simulink model "ALS"  (R2012b)
settings: Solver=ode1  StartTime=0.0  StopTime=200  FixedStep=0.05  RelTol=1e-3
undefined symbols (not defined in the file or in its folder): ACSP
libraries: simulink x2
settings Model: BufferReuse=off  Creator=jmbianni  LastModifiedBy=biannic
settings DataIOCC: InitialState=[]  LoadInitialState=on
settings OptimizationCC: InlineParams=on  BufferReuse=off
settings DebuggingCC: InitInArrayFormatMsg=none
settings CodeAppCC: CustomSymbolStrType=$N$R$M_T
settings GRTTargetCC: CodeReplacementLibrary=C89/C90 (ANSI)

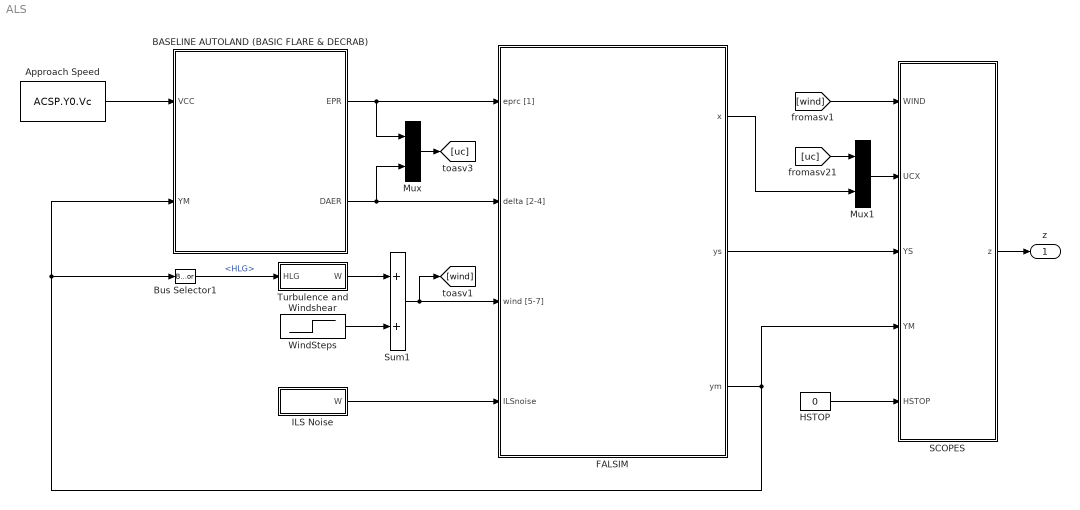
== system ALS ==
  Approach Speed : Constant  Value=ACSP.Y0.Vc
  BASELINE AUTOLAND (BASIC FLARE & DECRAB) : Subsystem
      mask Display:
      | image(imread('ALS.png'));
      | 
      | port_label('output', 1,'{\bf\fontsize{12}\delta_{TH}}', 'texmode','on');
      | port_label('output', 2,'{\bf\fontsize{12}\delta_{AER}}', 'texmode','on');
      | port_label('input', 1,'{\bf\fontsize{12}V_{APP}}', 'texmode','on');
      | port_label('input', 2,'{\bf\fontsize{12}YM}', 'texmode','on');
  Bus Selector1 : BusSelector  OutputSignals=HLG
  FALSIM : Subsystem
      mask Display:
      | image(imread('FALSIM.png'));
      | color('white');
      | disp('FINAL APPROACH & LANDING \n\n\n\n\n\n\n\n\n\n\n\n\n\n\n\n\n\n\n\n\n\n\n\n\n\n\n\n\n\n');
      | disp('SIMULATION MODEL \n\n\n\n\n\n\n\n\n\n\n\n\n\n\n\n\n\n\n\n\n\n\n\n\n\n\n\n');
      | 
      | color('red');
      | disp('http://w3.onera.fr/smac/ \n\n\n\n');
      | 
      | 
      | 
      | color('red');
      | %disp('{\bf\fontsize{12}SMAC TOOLS}', 'texmode','on');
      | 
      | color('yellow');
      | 
      | port_label('output', 1,'{\bf\fontsize{12}States}', 'texmode','on');
      | port_label('output', 2,'{\bf\fontsize{12}Non Measured Outputs}', 'texmode','on');
      | port_label('output', 3,'{\bf\fontsize{12}Measured Outputs}', 'texmode','on');
      | port_label('input', 1,'{\bf\fontsize{12}\delta_{TH}}', 'texmode','on');
      | port_label('input', 2,'{\bf\fontsize{12}\delta_A , \delta_E , \delta_R}', 'texmode','on');
      | port_label('input', 3,'{\bf\fontsize{12}W_x , W_y , W_z}', 'texmode','on');
      | port_label('input', 4,'{\bf\fontsize{12}W_{LOC} , W_{GLD}}', 'texmode','on');
  HSTOP : Constant  Value=0
  ILS Noise : Subsystem
  Mux : Mux  Inputs=2
  Mux1 : Mux  Inputs=2
  SCOPES : Subsystem
  Sum1 : Sum
  Turbulence and Windshear : Subsystem
  WindSteps : Step  Time=ACSP.TURBW.WindStepTime  After=ACSP.TURBW.WindStepMag  SampleTime=0
  z : Outport
  wires:
  BASELINE AUTOLAND (BASIC FLARE & DECRAB)/1(EPR) -> FALSIM/1(eprc [1]), Mux/1
  BASELINE AUTOLAND (BASIC FLARE & DECRAB)/2(DAER) -> FALSIM/2(delta [2-4]), Mux/2
  FALSIM/3(ym) -> SCOPES/4(YM), BASELINE AUTOLAND (BASIC FLARE & DECRAB)/2(YM), Bus Selector1/1
  Approach Speed/1 -> BASELINE AUTOLAND (BASIC FLARE & DECRAB)/1(VCC)
  SCOPES/1(z) -> z/1
  Mux/1 -> [uc]
  FALSIM/1(x) -> Mux1/2
  [uc] -> Mux1/1
  FALSIM/2(ys) -> SCOPES/3(YS)
  Mux1/1 -> SCOPES/2(UCX)
  HSTOP/1 -> SCOPES/5(HSTOP)
  Bus Selector1/1 -> Turbulence and Windshear/1(HLG)  "<HLG>"
  ILS Noise/1(W) -> FALSIM/4(ILSnoise)
  [wind] -> SCOPES/1(WIND)
  Sum1/1 -> FALSIM/3(wind [5-7]), [wind]
  Turbulence and Windshear/1(W) -> Sum1/1
  WindSteps/1 -> Sum1/2

== system ALS/BASELINE AUTOLAND (BASIC FLARE & DECRAB) ==
  VCC : Inport
  YM : Inport  Port=2
  DECRAB : Subsystem
  FLARE : Subsystem
  GLD  OUTER-LOOP : Subsystem
  HDEC : Constant  Value=ACSP.ALS.HDC
  HFLA : Constant  Value=ACSP.ALS.HFL
  LAT CONTROL : Subsystem
  LOC OUTER-LOOP : Subsystem
  LON CONTROL : Subsystem
  Mux : Mux  Inputs=2
  Switch DEC : Switch
  Switch FLA : Switch
  dth1 : Selector  InputPortWidth=4  IndexOptions=Index vector (dialog)  Indices=1  OutputSizes=1
  dth2 : Selector  InputPortWidth=4  IndexOptions=Index vector (dialog)  Indices=[3 2 4]  OutputSizes=1
  EPR : Outport
  DAER : Outport  Port=2
  wires:
  FLARE/2(dTH dE) -> Switch FLA/3
  FLARE/1(swF) -> Switch FLA/2
  HDEC/1 -> DECRAB/2(HDEC)
  dth2/1 -> DAER/1
  dth1/1 -> EPR/1
  Mux/1 -> dth2/1, dth1/1
  HFLA/1 -> FLARE/2(HFL)
  LON CONTROL/1(dTH  dE) -> Switch FLA/1, FLARE/1(dTHdE)
  Switch FLA/1 -> Mux/1
  DECRAB/1(swD) -> Switch DEC/2
  DECRAB/2(nyc,phic) -> Switch DEC/3
  Switch DEC/1 -> LAT CONTROL/2(nyc,phic)
  LOC OUTER-LOOP/1(nyc,phic) -> Switch DEC/1
  VCC/1 -> GLD  OUTER-LOOP/1(Vcc)
  LAT CONTROL/1(dA  dR) -> Mux/2
  GLD  OUTER-LOOP/1(vcc,vzc) -> LON CONTROL/1(vcc,vzc)
  YM/1 -> GLD  OUTER-LOOP/2(y), LON CONTROL/2(y), LAT CONTROL/1(y), FLARE/3(y), DECRAB/1(y), LOC OUTER-LOOP/1(y)

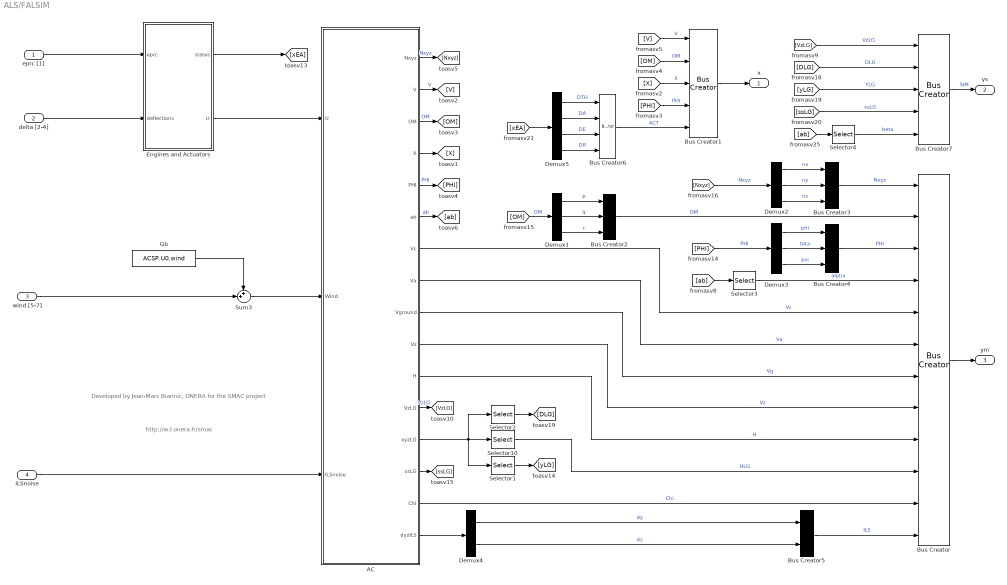
== system ALS/FALSIM ==
  note: http://w3.onera.fr/smac
  note: Developed by
      | Jean-Marc Biannic, ONERA
      | for the SMAC project
  eprc [1] : Inport
  delta [2-4] : Inport  Port=2  PortDimensions=3
  wind [5-7] : Inport  Port=3  PortDimensions=3
  ILSnoise : Inport  Port=4  PortDimensions=2
  AC : Subsystem
  Bus Creator : BusCreator  Inputs=12
  Bus Creator1 : BusCreator  Inputs=5
  Bus Creator2 : BusCreator  Inputs=3
  Bus Creator3 : BusCreator  Inputs=3
  Bus Creator4 : BusCreator  Inputs=3
  Bus Creator5 : BusCreator  Inputs=2
  Bus Creator6 : BusCreator
  Bus Creator7 : BusCreator  Inputs=5
  Demux1 : Demux  Outputs=3
  Demux2 : Demux  Outputs=3
  Demux3 : Demux  Outputs=3
  Demux4 : Demux  Outputs=2
  Demux5 : Demux
  Engines and Actuators : Subsystem
  Gb : Constant  Value=ACSP.U0.wind
  Selector1 : Selector  InputPortWidth=3  IndexOptions=Index vector (dialog)  Indices=2  OutputSizes=1
  Selector10 : Selector  InputPortWidth=3  IndexOptions=Index vector (dialog)  Indices=3  OutputSizes=1
  Selector2 : Selector  InputPortWidth=3  IndexOptions=Index vector (dialog)  Indices=1  OutputSizes=1
  Selector3 : Selector  InputPortWidth=2  IndexOptions=Index vector (dialog)  Indices=1  OutputSizes=1
  Selector4 : Selector  InputPortWidth=2  IndexOptions=Index vector (dialog)  Indices=2  OutputSizes=1
  Sum3 : Sum  Inputs=++|
  x : Outport
  ys : Outport  Port=2
  ym : Outport  Port=3
  wires:
  [VzLG] -> Bus Creator7/1  "VzLG"
  [DLG] -> Bus Creator7/2  "DLG"
  [yLG] -> Bus Creator7/3  "YLG"
  [ssLG] -> Bus Creator7/4  "ssLG"
  Selector4/1 -> Bus Creator7/5  "beta"
  delta [2-4]/1 -> Engines and Actuators/2(deflections)
  Bus Creator7/1 -> ys/1  "SIM"
  Bus Creator/1 -> ym/1
  Sum3/1 -> AC/2(Wind)
  Gb/1 -> Sum3/1
  ILSnoise/1 -> AC/3(ILSnoise)
  AC/11(H) -> Bus Creator/9  "H"
  AC/10(Vz) -> Bus Creator/8  "Vz"
  [ab] -> Selector4/1
  Bus Creator5/1 -> Bus Creator/12  "ILS"
  Bus Creator6/1 -> Bus Creator1/5  "ACT"
  [xEA] -> Demux5/1
  Demux5/4 -> Bus Creator6/4  "DR"
  Demux5/3 -> Bus Creator6/3  "DE"
  Demux5/2 -> Bus Creator6/2  "DA"
  Demux5/1 -> Bus Creator6/1  "DTH"
  Engines and Actuators/1(states) -> [xEA]
  Engines and Actuators/2(U) -> AC/1(U)
  eprc [1]/1 -> Engines and Actuators/1(eprc)
  Bus Creator1/1 -> x/1
  [PHI] -> Bus Creator1/4  "PHI"
  [X] -> Bus Creator1/3  "X"
  [OM] -> Bus Creator1/2  "OM"
  [V] -> Bus Creator1/1  "V"
  AC/12(VzLG) -> [VzLG]  "VzLG"
  AC/15(Chi) -> Bus Creator/11  "Chi"
  AC/9(Vground) -> Bus Creator/7  "Vg"
  AC/8(Va) -> Bus Creator/6  "Va"
  AC/7(Vc) -> Bus Creator/5  "Vc"
  AC/6(ab) -> [ab]  "ab"
  AC/5(PHI) -> [PHI]  "PHI"
  AC/4(X) -> [X]
  AC/3(OM) -> [OM]  "OM"
  AC/2(V) -> [V]  "V"
  AC/1(Nxyz) -> [Nxyz]  "Nxyz"
  Selector10/1 -> Bus Creator/10  "HLG"
  Selector2/1 -> [DLG]
  Demux4/2 -> Bus Creator5/2  "dz"
  Demux4/1 -> Bus Creator5/1  "dy"
  AC/16(dyzILS) -> Demux4/1
  AC/14(ssLG) -> [ssLG]
  Selector1/1 -> [yLG]
  AC/13(xyzLG) -> Selector2/1, Selector10/1, Selector1/1
  Bus Creator4/1 -> Bus Creator/3  "PHI"
  [PHI] -> Demux3/1  "PHI"
  Demux3/1 -> Bus Creator4/1  "phi"
  Demux3/2 -> Bus Creator4/2  "teta"
  Demux3/3 -> Bus Creator4/3  "psi"
  Bus Creator3/1 -> Bus Creator/1  "Nxyz"
  [Nxyz] -> Demux2/1  "Nxyz"
  Demux2/1 -> Bus Creator3/1  "nx"
  Demux2/2 -> Bus Creator3/2  "ny"
  Demux2/3 -> Bus Creator3/3  "nz"
  [OM] -> Demux1/1  "OM"
  Demux1/1 -> Bus Creator2/1  "p"
  Demux1/2 -> Bus Creator2/2  "q"
  Demux1/3 -> Bus Creator2/3  "r"
  Bus Creator2/1 -> Bus Creator/2  "OM"
  [ab] -> Selector3/1
  Selector3/1 -> Bus Creator/4  "alpha"
  wind [5-7]/1 -> Sum3/2

== system ALS/ILS Noise ==
  Mux : Mux  Inputs=2
  Random Number : RandomNumber  Seed=ACSP.NOISE.seedLOC  SampleTime=0.05
  Random Number3 : RandomNumber  Seed=ACSP.NOISE.seedGLD  SampleTime=0.05
  Sum12 : Sum  Inputs=++|
  bias : Constant  Value=ACSP.NOISE.devLOC
  sigGLD : Gain  Gain=ACSP.NOISE.sigGLD
  sigLOC : Gain  Gain=ACSP.NOISE.sigLOC
  srqt(2*tau/ts)*1/(1+tau.s) : TransferFcn  Numerator=[4.5]  Denominator=[0.5 1]
  srqt(2*tau/ts)*1/(1+tau.s)1 : TransferFcn  Numerator=[4.5]  Denominator=[0.5 1]
  W : Outport
  wires:
  bias/1 -> Sum12/1
  Sum12/1 -> Mux/1
  sigLOC/1 -> Sum12/2
  sigGLD/1 -> Mux/2
  srqt(2*tau/ts)*1/(1+tau.s)/1 -> sigLOC/1
  Random Number3/1 -> srqt(2*tau/ts)*1/(1+tau.s)1/1
  Random Number/1 -> srqt(2*tau/ts)*1/(1+tau.s)/1
  Mux/1 -> W/1
  srqt(2*tau/ts)*1/(1+tau.s)1/1 -> sigGLD/1

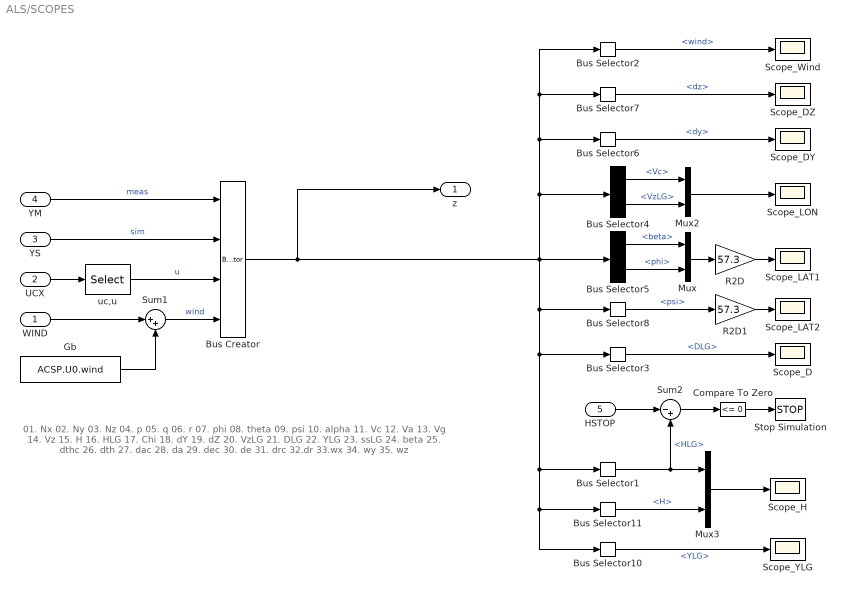
== system ALS/SCOPES ==
  note: 01. Nx       02. Ny        03. Nz         04. p         05. q         06. r        07. phi         08. theta           09. psi
      | 10. alpha        11. Vc       12. Va      13. Vg       14. Vz        15. H        16. HLG       17. Chi     18. dY
      | 19. dZ     20. VzLG         21. DLG     22. YLG    23. ssLG      24. beta       25. dthc      26. dth
      |  27. dac        28. da          29. dec          30. de          31.  drc        32.dr        33.wx      34. wy    35. wz
  WIND : Inport
  UCX : Inport  Port=2
  YS : Inport  Port=3
  YM : Inport  Port=4
  HSTOP : Inport  Port=5
  Bus Creator : BusCreator
  Bus Selector1 : BusSelector  OutputSignals=meas.HLG
  Bus Selector10 : BusSelector  OutputSignals=sim.YLG
  Bus Selector11 : BusSelector  OutputSignals=meas.H
  Bus Selector2 : BusSelector  OutputSignals=wind
  Bus Selector3 : BusSelector  OutputSignals=sim.DLG
  Bus Selector4 : BusSelector  OutputSignals=meas.Vc,sim.VzLG
  Bus Selector5 : BusSelector  OutputSignals=sim.beta,meas.PHI.phi
  Bus Selector6 : BusSelector  OutputSignals=meas.ILS.dy
  Bus Selector7 : BusSelector  OutputSignals=meas.ILS.dz
  Bus Selector8 : BusSelector  OutputSignals=meas.PHI.psi
  Compare To Zero : simulink/Logic and Bit Operations/Compare To Zero  relop=<=  OutDataTypeStr=boolean
  Gb : Constant  Value=ACSP.U0.wind
  Mux : Mux  Inputs=2
  Mux2 : Mux  Inputs=2
  Mux3 : Mux  Inputs=2
  R2D : Gain  Gain=57.3
  R2D1 : Gain  Gain=57.3
  Scope_D : Scope
      settings: SaveName=ScopeData9
  Scope_DY : Scope
  Scope_DZ : Scope
      settings: SaveName=ScopeData2  Decimation=2
  Scope_H : Scope
      settings: SaveName=ScopeData3  Decimation=2
  Scope_LAT1 : Scope
      settings: SaveName=ScopeData4
  Scope_LAT2 : Scope
  Scope_LON : Scope
      settings: SaveName=ScopeData5
  Scope_Wind : Scope
      settings: SaveName=ScopeData8  Decimation=2
  Scope_YLG : Scope
      settings: YMin=2.5  YMax=22.5  SaveName=ScopeData6  Decimation=2
  Stop Simulation : Stop
  Sum1 : Sum  Inputs=|++
  Sum2 : Sum  Inputs=|-+
  uc,u : Selector  InputPortWidth=20  IndexOptions=Index vector (dialog)  Indices=[1 17 2 18 3 19 4 20]  OutputSizes=1
  z : Outport
  wires:
  Bus Selector10/1 -> Scope_YLG/1  "<YLG>"
  Mux3/1 -> Scope_H/1
  Bus Selector3/1 -> Scope_D/1  "<DLG>"
  R2D1/1 -> Scope_LAT2/1
  Bus Selector8/1 -> R2D1/1  "<psi>"
  R2D/1 -> Scope_LAT1/1
  Mux/1 -> R2D/1
  Mux2/1 -> Scope_LON/1
  Bus Selector4/2 -> Mux2/2  "<VzLG>"
  Bus Selector4/1 -> Mux2/1  "<Vc>"
  YM/1 -> Bus Creator/1  "meas"
  Bus Selector7/1 -> Scope_DZ/1  "<dz>"
  Bus Selector6/1 -> Scope_DY/1  "<dy>"
  YS/1 -> Bus Creator/2  "sim"
  Bus Selector1/1 -> Sum2/2, Mux3/1  "<HLG>"
  Bus Selector11/1 -> Mux3/2  "<H>"
  Bus Creator/1 -> Bus Selector2/1, Bus Selector7/1, Bus Selector6/1, Bus Selector4/1, Bus Selector10/1, Bus Selector11/1, Bus Selector1/1, Bus Selector3/1, Bus Selector8/1, Bus Selector5/1, z/1
  uc,u/1 -> Bus Creator/3  "u"
  Bus Selector5/2 -> Mux/2  "<phi>"
  UCX/1 -> uc,u/1
  Bus Selector5/1 -> Mux/1  "<beta>"
  Compare To Zero/1 -> Stop Simulation/1
  Sum2/1 -> Compare To Zero/1
  HSTOP/1 -> Sum2/1
  WIND/1 -> Sum1/1
  Gb/1 -> Sum1/2
  Sum1/1 -> Bus Creator/4  "wind"
  Bus Selector2/1 -> Scope_Wind/1  "<wind>"

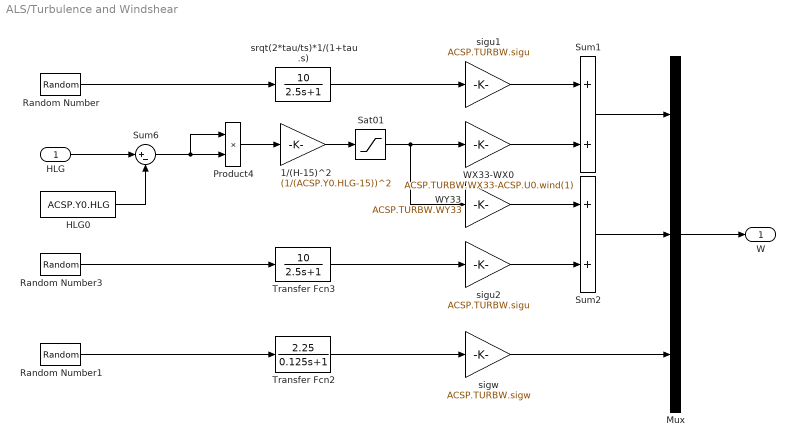
== system ALS/Turbulence and Windshear ==
  HLG : Inport
  1/(H-15)^2 : Gain  Gain=(1/(ACSP.Y0.HLG-15))^2
  HLG0 : Constant  Value=ACSP.Y0.HLG
  Mux : Mux  Inputs=3
  Product4 : Product  SaturateOnIntegerOverflow=on  RndMeth=Zero  InputSameDT=on  OutDataTypeStr=Inherit: Same as first input
  Random Number : RandomNumber  Seed=ACSP.TURBW.seedwx  SampleTime=0.05
  Random Number1 : RandomNumber  Seed=ACSP.TURBW.seedwz  SampleTime=0.05
  Random Number3 : RandomNumber  Seed=ACSP.TURBW.seedwy  SampleTime=0.05
  Sat01 : Saturate  UpperLimit=1  LowerLimit=0
  Sum1 : Sum
  Sum2 : Sum
  Sum6 : Sum  Inputs=|+-
  Transfer Fcn2 : TransferFcn  Numerator=[2.25]  Denominator=[0.125 1]
  Transfer Fcn3 : TransferFcn  Numerator=[10]  Denominator=[2.5 1]
  WX33-WX0 : Gain  Gain=ACSP.TURBW.WX33-ACSP.U0.wind(1)
  WY33 : Gain  Gain=ACSP.TURBW.WY33
  sigu1 : Gain  Gain=ACSP.TURBW.sigu
  sigu2 : Gain  Gain=ACSP.TURBW.sigu
  sigw : Gain  Gain=ACSP.TURBW.sigw
  srqt(2*tau/ts)*1/(1+tau.s) : TransferFcn  Numerator=[10]  Denominator=[2.5 1]
  W : Outport
  wires:
  sigu2/1 -> Sum2/2
  sigu1/1 -> Sum1/1
  Random Number1/1 -> Transfer Fcn2/1
  Transfer Fcn2/1 -> sigw/1
  Mux/1 -> W/1
  HLG/1 -> Sum6/1
  HLG0/1 -> Sum6/2
  Sum6/1 -> Product4/1, Product4/2
  Product4/1 -> 1/(H-15)^2/1
  1/(H-15)^2/1 -> Sat01/1
  Sat01/1 -> WY33/1, WX33-WX0/1
  srqt(2*tau/ts)*1/(1+tau.s)/1 -> sigu1/1
  Transfer Fcn3/1 -> sigu2/1
  sigw/1 -> Mux/3
  WX33-WX0/1 -> Sum1/2
  Sum2/1 -> Mux/2
  WY33/1 -> Sum2/1
  Sum1/1 -> Mux/1
  Random Number3/1 -> Transfer Fcn3/1
  Random Number/1 -> srqt(2*tau/ts)*1/(1+tau.s)/1

== system ALS/BASELINE AUTOLAND (BASIC FLARE & DECRAB)/DECRAB ==
  y : Inport
  HDEC : Inport  Port=2
  Bus Selector1 : BusSelector  OutputSignals=PHI.psi
  Bus Selector2 : BusSelector  OutputSignals=HLG
  Dec Gain : Gain  Gain=5
  Mux1 : Mux  Inputs=2
  PHICD : Constant  Value=0
  RL : RateLimiter  RisingSlewLimit=0  FallingSlewLimit=-10  SampleTimeMode=inherited
  Sum3 : Sum  Inputs=-+|
  swD : Outport
  nyc,phic : Outport  Port=2
  wires:
  Dec Gain/1 -> Mux1/1
  Mux1/1 -> nyc,phic/1
  PHICD/1 -> Mux1/2
  Bus Selector1/1 -> Dec Gain/1  "<psi>"
  HDEC/1 -> Sum3/1
  Bus Selector2/1 -> Sum3/2  "<HLG>"
  y/1 -> Bus Selector2/1, Bus Selector1/1
  Sum3/1 -> RL/1
  RL/1 -> swD/1

== system ALS/BASELINE AUTOLAND (BASIC FLARE & DECRAB)/FLARE ==
  dTHdE : Inport
  HFL : Inport  Port=2
  y : Inport  Port=3
  Bus Selector1 : BusSelector  OutputSignals=Vz
  Bus Selector2 : BusSelector  OutputSignals=HLG
  Freeze : Subsystem
  Gain : Gain  Gain=-0.018
  Mux1 : Mux  Inputs=2
  RL : RateLimiter  RisingSlewLimit=0  FallingSlewLimit=-10  SampleTimeMode=inherited
  Sum1 : Sum  Inputs=|+-
  Sum2 : Sum  Inputs=|+-
  Sum4 : Sum  Inputs=|+-
  de : Selector  InputPortWidth=2  IndexOptions=Index vector (dialog)  Indices=2  OutputSizes=1
  dth : Selector  InputPortWidth=2  IndexOptions=Index vector (dialog)  Indices=1  OutputSizes=1
  vzt1 : Constant  Value=-0.75
  swF : Outport
  dTH dE : Outport  Port=2
  wires:
  Gain/1 -> Sum4/2
  Sum2/1 -> Gain/1
  vzt1/1 -> Sum2/2
  Bus Selector1/1 -> Sum2/1  "<Vz>"
  RL/1 -> swF/1, Freeze/2(swF)
  dTHdE/1 -> Freeze/1(w)
  Mux1/1 -> dTH dE/1
  Sum4/1 -> Mux1/2
  de/1 -> Sum4/1
  dth/1 -> Mux1/1
  Freeze/1(z) -> dth/1, de/1
  HFL/1 -> Sum1/2
  Bus Selector2/1 -> Sum1/1  "<HLG>"
  Sum1/1 -> RL/1
  y/1 -> Bus Selector2/1, Bus Selector1/1

== system ALS/BASELINE AUTOLAND (BASIC FLARE & DECRAB)/GLD  OUTER-LOOP ==
  Vcc : Inport
  y : Inport  Port=2
  Bus Selector2 : BusSelector  OutputSignals=ILS.dz
  KGLD : Gain  Gain=ACSP.ALS.kpGLD
  Mux1 : Mux  Inputs=2
  Saturation : Saturate  UpperLimit=15  LowerLimit=-15
  Sum4 : Sum  Inputs=-+|
  Vc0 : Constant  Value=ACSP.Y0.Vc
  sign : Gain  Gain=-1
  vcc,vzc : Outport
  wires:
  Bus Selector2/1 -> Saturation/1  "<dz>"
  Mux1/1 -> vcc,vzc/1
  Saturation/1 -> KGLD/1
  Vc0/1 -> Sum4/1
  Vcc/1 -> Sum4/2
  Sum4/1 -> Mux1/1
  sign/1 -> Mux1/2
  KGLD/1 -> sign/1
  y/1 -> Bus Selector2/1

== system ALS/BASELINE AUTOLAND (BASIC FLARE & DECRAB)/LAT CONTROL ==
  y : Inport
  nyc,phic : Inport  Port=2
  HLAT : Gain  Gain=ACSP.ALS.HLAT  Multiplication=Matrix(K*u)
  IntVc : Integrator
  KLAT : Gain  Gain=ACSP.ALS.KLAT  Multiplication=Matrix(K*u)
  Mux : Mux  Inputs=2
  NyPRphi : BusSelector  OutputSignals=Nxyz.ny,OM.p,OM.r,PHI.phi  OutputAsBus=on
  NyPRphi0 : Subsystem
  Sum1 : Sum  Inputs=|+-
  Sum2 : Sum  Inputs=++|
  Sum3 : Sum  Inputs=-+|
  ny,phi : Selector  InputPortWidth=4  IndexOptions=Index vector (dialog)  Indices=[1 4]  OutputSizes=1
  dA  dR : Outport
  wires:
  NyPRphi0/1(y0) -> Sum3/1
  NyPRphi/1 -> Sum3/2
  HLAT/1 -> Sum2/1
  Sum2/1 -> dA  dR/1
  KLAT/1 -> Sum2/2
  ny,phi/1 -> Sum1/2
  Sum3/1 -> Mux/2, ny,phi/1
  y/1 -> NyPRphi/1
  Sum1/1 -> IntVc/1
  nyc,phic/1 -> HLAT/1, Sum1/1
  IntVc/1 -> Mux/1
  Mux/1 -> KLAT/1

== system ALS/BASELINE AUTOLAND (BASIC FLARE & DECRAB)/LOC OUTER-LOOP ==
  y : Inport
  Bus Selector : BusSelector  OutputSignals=Chi
  Bus Selector1 : BusSelector  OutputSignals=Vg
  Bus Selector2 : BusSelector  OutputSignals=ILS.dy
  Mux1 : Mux  Inputs=2
  NYCA : Constant  Value=0
  Product1 : Product  RndMeth=Zero
  Sum4 : Sum  Inputs=|++
  kdLOC : Gain  Gain=ACSP.ALS.kdLOC
  kpLOC : Gain  Gain=ACSP.ALS.kpLOC
  sign : Gain  Gain=-1
  nyc,phic : Outport
  wires:
  Mux1/1 -> nyc,phic/1
  sign/1 -> Mux1/2
  NYCA/1 -> Mux1/1
  kdLOC/1 -> Sum4/1
  kpLOC/1 -> Sum4/2
  Sum4/1 -> sign/1
  Bus Selector/1 -> Product1/1  "<Chi>"
  Bus Selector1/1 -> Product1/2  "<Vg>"
  y/1 -> Bus Selector2/1, Bus Selector1/1, Bus Selector/1
  Bus Selector2/1 -> kpLOC/1  "<dy>"
  Product1/1 -> kdLOC/1

== system ALS/BASELINE AUTOLAND (BASIC FLARE & DECRAB)/LON CONTROL ==
  vcc,vzc : Inport
  y : Inport  Port=2
  Bus Selector1 : BusSelector  OutputSignals=Vc,Vz,OM.q,Nxyz.nz  OutputAsBus=on
  HLON : Gain  Gain=ACSP.ALS.HLON  Multiplication=Matrix(K*u)
  IntVc : Integrator
  KLON : Gain  Gain=ACSP.ALS.KLON  Multiplication=Matrix(K*u)
  Mux : Mux  Inputs=2
  Sum1 : Sum  Inputs=|+-
  Sum2 : Sum  Inputs=++|
  Sum3 : Sum  Inputs=-+|
  VcVzQNZ0 : Subsystem
  vc,vz : Selector  InputPortWidth=4  IndexOptions=Index vector (dialog)  Indices=[1 2]  OutputSizes=1
  dTH  dE : Outport
  wires:
  VcVzQNZ0/1(y0) -> Sum3/1
  Bus Selector1/1 -> Sum3/2
  HLON/1 -> Sum2/1
  Sum2/1 -> dTH  dE/1
  KLON/1 -> Sum2/2
  Sum3/1 -> vc,vz/1, Mux/2
  Mux/1 -> KLON/1
  y/1 -> Bus Selector1/1
  vc,vz/1 -> Sum1/2
  Sum1/1 -> IntVc/1
  vcc,vzc/1 -> Sum1/1, HLON/1
  IntVc/1 -> Mux/1

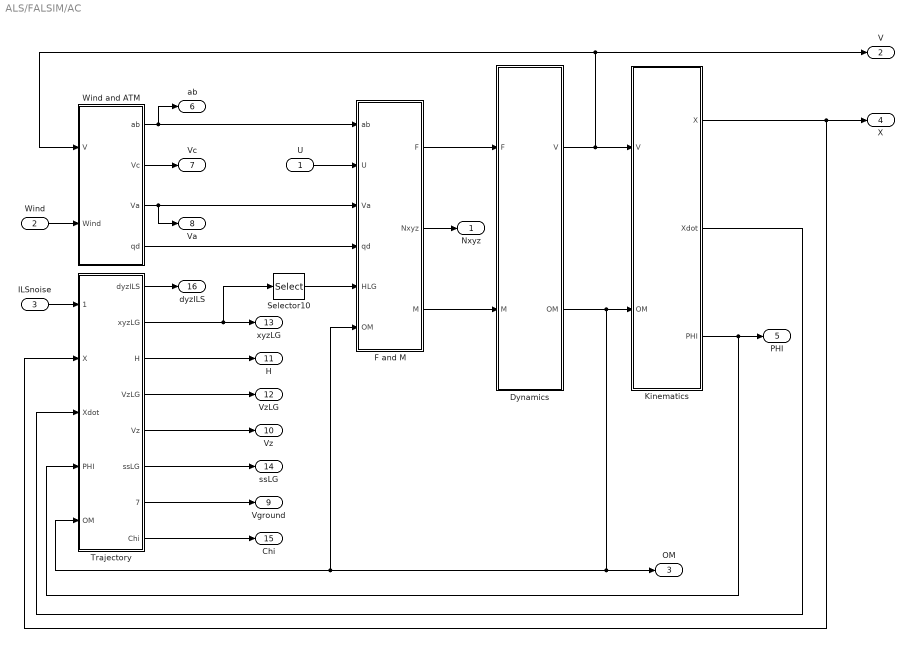
== system ALS/FALSIM/AC ==
  U : Inport
  Wind : Inport  Port=2  PortDimensions=3
  ILSnoise : Inport  Port=3  PortDimensions=2
  Dynamics : Subsystem
  F and M : Subsystem
  Kinematics : Subsystem
  Selector10 : Selector  InputPortWidth=3  IndexOptions=Index vector (dialog)  Indices=3  OutputSizes=1
  Trajectory : Subsystem
  Wind and ATM : Subsystem
  Nxyz : Outport
  V : Outport  Port=2
  OM : Outport  Port=3
  X : Outport  Port=4
  PHI : Outport  Port=5
  ab : Outport  Port=6
  Vc : Outport  Port=7
  Va : Outport  Port=8
  Vground : Outport  Port=9
  Vz : Outport  Port=10
  H : Outport  Port=11
  VzLG : Outport  Port=12
  xyzLG : Outport  Port=13
  ssLG : Outport  Port=14
  Chi : Outport  Port=15
  dyzILS : Outport  Port=16
  wires:
  ILSnoise/1 -> Trajectory/1(ILSnoise)
  Trajectory/5(Vz) -> Vz/1
  Trajectory/3(H) -> H/1
  Trajectory/6(ssLG) -> ssLG/1
  Trajectory/7(Vground) -> Vground/1
  Trajectory/8(Chi) -> Chi/1
  Trajectory/4(VzLG) -> VzLG/1
  Trajectory/1(dyzILS) -> dyzILS/1
  Trajectory/2(xyzLG) -> Selector10/1, xyzLG/1
  Selector10/1 -> F and M/5(HLG)
  Kinematics/1(X) -> Trajectory/2(X), X/1
  F and M/3(M) -> Dynamics/2(M)
  F and M/1(F) -> Dynamics/1(F)
  Dynamics/1(V) -> Wind and ATM/1(V), V/1, Kinematics/1(V)
  Dynamics/2(OM) -> OM/1, Trajectory/5(OM), F and M/6(OM), Kinematics/2(OM)
  Kinematics/3(PHI) -> PHI/1, Trajectory/4(PHI)
  Kinematics/2(Xdot) -> Trajectory/3(Xdot)
  Wind/1 -> Wind and ATM/2(Wind)
  Wind and ATM/2(Vc) -> Vc/1
  Wind and ATM/3(Va) -> Va/1, F and M/3(Va)
  Wind and ATM/4(qd) -> F and M/4(qd)
  U/1 -> F and M/2(U)
  Wind and ATM/1(ab) -> ab/1, F and M/1(ab)
  F and M/2(Nxyz) -> Nxyz/1

== system ALS/FALSIM/Engines and Actuators ==
  eprc : Inport
  deflections : Inport  Port=2
  Actuators : Subsystem
  Engines : Subsystem
  Mux : Mux  Inputs=2
  Mux1 : Mux  Inputs=2
  Sum3 : Sum  Inputs=|++
  delta0 : Constant  Value=ACSP.U0.delta
  epr0 : Constant  Value=ACSP.U0.epr
  states : Outport
  U : Outport  Port=2
  wires:
  delta0/1 -> Sum3/2
  Sum3/1 -> Mux/2
  Mux1/1 -> states/1
  Engines/2(epr) -> Mux1/1  "EPR"
  Mux/1 -> U/1
  epr0/1 -> Engines/1(epr0)
  deflections/1 -> Actuators/1(deltac)
  eprc/1 -> Engines/2(eprc)
  Engines/1(TH) -> Mux/1
  Actuators/1(delta) -> Mux1/2, Sum3/1

== system ALS/BASELINE AUTOLAND (BASIC FLARE & DECRAB)/FLARE/Freeze ==
  w : Inport
  swF : Inport  Port=2
  Compare To Zero : simulink/Logic and Bit Operations/Compare To Zero  relop=>=  OutDataTypeStr=boolean
  Integrator : Integrator
  Product : Product  RndMeth=Zero
  Product1 : Product  Inputs=/*  RndMeth=Zero
  Sum1 : Sum  Inputs=|+-
  Sum2 : Sum  Inputs=|-+
  "[0.1 2]" : Saturate  UpperLimit=2  LowerLimit=0.1
  vzt1 : Constant  Value=15
  z : Outport
  wires:
  Sum1/1 -> Product/2
  w/1 -> Sum1/1
  Integrator/1 -> z/1, Sum1/2
  vzt1/1 -> Sum2/1
  Sum2/1 -> "[0.1 2]"/1
  "[0.1 2]"/1 -> Product1/1
  Product/1 -> Product1/2
  Product1/1 -> Integrator/1
  Compare To Zero/1 -> Product/1
  swF/1 -> Compare To Zero/1, Sum2/2

== system ALS/BASELINE AUTOLAND (BASIC FLARE & DECRAB)/LAT CONTROL/NyPRphi0 ==
  Mux1 : Mux
  Ny0 : Constant  Value=ACSP.Y0.Ny
  p0 : Constant  Value=ACSP.Y0.p
  phi0 : Constant  Value=ACSP.Y0.phi
  r0 : Constant  Value=ACSP.Y0.r
  y0 : Outport
  wires:
  Ny0/1 -> Mux1/1
  Mux1/1 -> y0/1
  r0/1 -> Mux1/3
  p0/1 -> Mux1/2
  phi0/1 -> Mux1/4

== system ALS/BASELINE AUTOLAND (BASIC FLARE & DECRAB)/LON CONTROL/VcVzQNZ0 ==
  Mux1 : Mux
  Nz0 : Constant  Value=ACSP.Y0.Nz
  Vc0 : Constant  Value=ACSP.Y0.Vc
  Vz0 : Constant  Value=ACSP.Y0.Vz
  q0 : Constant  Value=ACSP.Y0.q
  y0 : Outport
  wires:
  Vc0/1 -> Mux1/1
  Mux1/1 -> y0/1
  q0/1 -> Mux1/3
  Vz0/1 -> Mux1/2
  Nz0/1 -> Mux1/4

== system ALS/FALSIM/AC/Dynamics ==
  note: M = I*OMdot + OM x (I*OM)
  note: F =mass*(Vdot + OM x V)
  F : Inport
  M : Inport  Port=2
  CP1 : Subsystem
      mask Display:
      | fprintf('CROSS \n PRODUCT');
      | color('red');
      | fprintf('\n\n');
      | fprintf(' \n \n \n z=x^y');
      | %text(3,1,'PRODUCT');
      | %text(5,1,'z=x^y');
  CP2 : Subsystem
      mask Display:
      | fprintf('CROSS \n PRODUCT');
      | color('red');
      | fprintf('\n\n');
      | fprintf(' \n \n \n z=x^y');
      | %text(3,1,'PRODUCT');
      | %text(5,1,'z=x^y');
  Inertia : Gain  Gain=ACSP.MIG.I  Multiplication=Matrix(K*u)
  Inertia^-1 : Gain  Gain=ACSP.MIG.J  Multiplication=Matrix(K*u)
  Int_OM : Integrator  InitialCondition=ACSP.X0.OM  ContinuousStateAttributes='OM'
  Int_V : Integrator  InitialCondition=ACSP.X0.V  ContinuousStateAttributes='V'
  Mass^-1 : Gain  Gain=1/ACSP.MIG.mass
  Sum : Sum  Inputs=|+-
  Sum1 : Sum  Inputs=-+|
  V : Outport
  OM : Outport  Port=2
  wires:
  Inertia/1 -> CP1/2(y)
  Mass^-1/1 -> Sum1/2
  CP1/1(z) -> Sum/2
  CP2/1(z) -> Sum1/1
  Int_OM/1 -> OM/1, CP2/1(x), Inertia/1, CP1/1(x)
  F/1 -> Mass^-1/1
  Inertia^-1/1 -> Int_OM/1
  M/1 -> Sum/1
  Sum/1 -> Inertia^-1/1
  Sum1/1 -> Int_V/1
  Int_V/1 -> V/1, CP2/2(y)

== system ALS/FALSIM/AC/F and M ==
  ab : Inport
  U : Inport  Port=2
  Va : Inport  Port=3
  qd : Inport  Port=4
  HLG : Inport  Port=5
  OM : Inport  Port=6
  Bus Creator : BusCreator  Inputs=10
  Demux1 : Demux  Outputs=3
  Demux2 : Demux  Outputs=3
  Demux3 : Demux  Outputs=2
  Forces : Subsystem
  Moments : Subsystem
  S : Gain  Gain=ACSP.MIG.Sref
  Selector : Selector  InputPortWidth=4  IndexOptions=Index vector (dialog)  Indices=[2 3 4]  OutputSizes=1
  Selector1 : Selector  InputPortWidth=4  IndexOptions=Index vector (dialog)  Indices=[1]  OutputSizes=1
  F : Outport
  Nxyz : Outport  Port=2
  M : Outport  Port=3
  wires:
  ab/1 -> Demux3/1  "alpha"
  Demux3/1 -> Bus Creator/1  "alpha"
  qd/1 -> S/1
  OM/1 -> Demux1/1
  HLG/1 -> Bus Creator/7  "Hlg"
  Va/1 -> Bus Creator/6  "Va"
  Demux2/1 -> Bus Creator/8  "da"
  Demux2/2 -> Bus Creator/9  "de"
  Demux2/3 -> Bus Creator/10  "dr"
  Demux3/2 -> Bus Creator/2  "beta"
  Demux1/3 -> Bus Creator/5  "r"
  Demux1/2 -> Bus Creator/4  "q"
  Demux1/1 -> Bus Creator/3  "p"
  Bus Creator/1 -> Forces/1(E), Moments/1(E)
  Moments/1(M) -> M/1
  Selector/1 -> Demux2/1
  U/1 -> Selector1/1, Selector/1
  Forces/1(Fa) -> Moments/2(Fa)
  S/1 -> Forces/3(qS), Moments/3(qS)
  Forces/2(F) -> F/1
  Selector1/1 -> Forces/2(TH), Moments/4(TH)
  Forces/3(Nxyz) -> Nxyz/1

== system ALS/FALSIM/AC/Kinematics ==
  V : Inport
  OM : Inport  Port=2
  Int_PHI : Integrator  InitialCondition=ACSP.X0.PHI  ContinuousStateAttributes='PHI'
  Int_X : Integrator  InitialCondition=ACSP.X0.X  ContinuousStateAttributes='X'
  R(PHI) : Subsystem
      mask Display:
      | fprintf('MATRIX \n PRODUCT');
      | color('red');
      | fprintf('\n\n');
      | fprintf(' \n \n \n z=M(x)*y');
  Rotations and transformations matrices : Subsystem
  T(PHI) : Subsystem
      mask Display:
      | fprintf('MATRIX \n PRODUCT');
      | color('red');
      | fprintf('\n\n');
      | fprintf(' \n \n \n z=M(x)*y');
  X : Outport
  Xdot : Outport  Port=2
  PHI : Outport  Port=3
  tag scope: RV2B=global
  wires:
  OM/1 -> T(PHI)/2(y)
  V/1 -> R(PHI)/2(y)
  R(PHI)/1(z) -> Int_X/1, Xdot/1
  Int_PHI/1 -> Rotations and transformations matrices/1(PHI), PHI/1
  Int_X/1 -> X/1
  Rotations and transformations matrices/3(RB2V) -> R(PHI)/1(x)
  Rotations and transformations matrices/1(TPHI) -> T(PHI)/1(x)
  Rotations and transformations matrices/2(RV2B) -> [RV2B]
  T(PHI)/1(z) -> Int_PHI/1

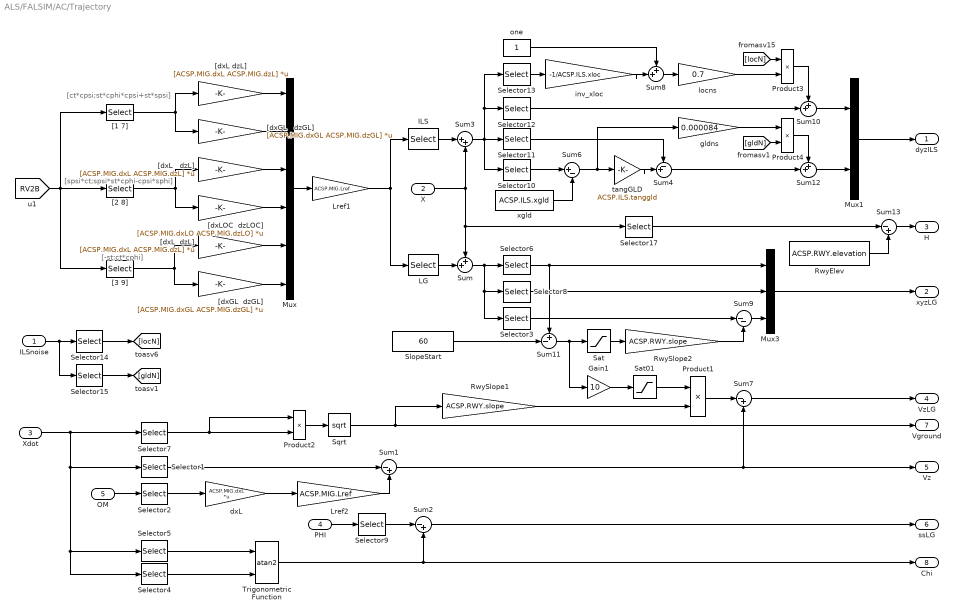
== system ALS/FALSIM/AC/Trajectory ==
  note: [spsi*ct;spsi*st*cphi-cpsi*sphi]
  note: [ct*cpsi;st*cphi*cpsi+st*spsi]
  note: [-st;ct*cphi]
  ILSnoise : Inport
  X : Inport  Port=2
  Xdot : Inport  Port=3
  PHI : Inport  Port=4
  OM : Inport  Port=5
  Gain1 : Gain  Gain=10
  ILS : Selector  InputPortWidth=6  IndexOptions=Index vector (dialog)  Indices=[2 4 6]  OutputSizes=1
  LG : Selector  InputPortWidth=6  IndexOptions=Index vector (dialog)  Indices=[1 3 5]  OutputSizes=1
  Lref1 : Gain  Gain=ACSP.MIG.Lref
  Lref2 : Gain  Gain=ACSP.MIG.Lref
  Mux : Mux  Inputs=6
  Mux1 : Mux  Inputs=2
  Mux3 : Mux  Inputs=3
  Product{1..4} (4 alike) : Product  SaturateOnIntegerOverflow=on  RndMeth=Zero  InputSameDT=on  OutDataTypeStr=Inherit: Same as first input
  RwyElev : Constant  Value=ACSP.RWY.elevation
  RwySlope1 : Gain  Gain=ACSP.RWY.slope
  RwySlope2 : Gain  Gain=ACSP.RWY.slope
  Sat : Saturate  UpperLimit=1000  LowerLimit=0
  Sat01 : Saturate  UpperLimit=1  LowerLimit=0
  Selector{1,3,9,11,17} (5 alike) : Selector  InputPortWidth=3  IndexOptions=Index vector (dialog)  Indices=3  OutputSizes=1
  Selector{4,6..7,10,13} (5 alike) : Selector  InputPortWidth=3  IndexOptions=Index vector (dialog)  Indices=1  OutputSizes=1
  Selector{2,5,8,12} (4 alike) : Selector  InputPortWidth=3  IndexOptions=Index vector (dialog)  Indices=2  OutputSizes=1
  Selector14 : Selector  InputPortWidth=2  IndexOptions=Index vector (dialog)  Indices=1  OutputSizes=1
  Selector15 : Selector  InputPortWidth=2  IndexOptions=Index vector (dialog)  Indices=2  OutputSizes=1
  SlopeStart : Constant  Value=60
  Sqrt : Sqrt  SaturateOnIntegerOverflow=on
  Sum{,8,10,12} (4 alike) : Sum  Inputs=++|
  Sum{1..2,7,13} (4 alike) : Sum  Inputs=|-+
  Sum11 : Sum  Inputs=+-|
  Sum3 : Sum  Inputs=|++
  Sum4 : Sum  Inputs=-+|
  Sum6 : Sum  Inputs=|+-
  Sum9 : Sum  Inputs=|--
  Trigonometric Function : Trigonometry  Operator=atan2
  "[1 7]" : Selector  InputPortWidth=9  IndexOptions=Index vector (dialog)  Indices=[1 7]  OutputSizes=1
  "[2 8]" : Selector  InputPortWidth=9  IndexOptions=Index vector (dialog)  Indices=[2 8]  OutputSizes=1
  "[3 9]" : Selector  InputPortWidth=9  IndexOptions=Index vector (dialog)  Indices=[3 9]  OutputSizes=1
  "[dxGL   dzGL]" : Gain  Gain=[ACSP.MIG.dxGL ACSP.MIG.dzGL]  Multiplication=Matrix(K*u)
  "[dxGL  dzGL]" : Gain  Gain=[ACSP.MIG.dxGL ACSP.MIG.dzGL]  Multiplication=Matrix(K*u)
  "[dxL   dzL]" : Gain  Gain=[ACSP.MIG.dxL ACSP.MIG.dzL]  Multiplication=Matrix(K*u)
  "[dxL  dzL]" : Gain  Gain=[ACSP.MIG.dxL ACSP.MIG.dzL]  Multiplication=Matrix(K*u)
  "[dxL dzL]" : Gain  Gain=[ACSP.MIG.dxL ACSP.MIG.dzL]  Multiplication=Matrix(K*u)
  "[dxLOC  dzLOC]" : Gain  Gain=[ACSP.MIG.dxLO ACSP.MIG.dzLO]  Multiplication=Matrix(K*u)
  dxL : Gain  Gain=ACSP.MIG.dxL  Multiplication=Matrix(K*u)
  gldns : Gain  Gain=0.000084
  inv_xloc : Gain  Gain=-1/ACSP.ILS.xloc
  locns : Gain  Gain=0.7
  one : Constant
  tangGLD : Gain  Gain=ACSP.ILS.tanggld
  xgld : Constant  Value=ACSP.ILS.xgld
  dyzILS : Outport
  xyzLG : Outport  Port=2
  H : Outport  Port=3
  VzLG : Outport  Port=4
  Vz : Outport  Port=5
  ssLG : Outport  Port=6
  Vground : Outport  Port=7
  Chi : Outport  Port=8
  wires:
  Selector3/1 -> Sum9/1
  RwySlope2/1 -> Sum9/2
  Sum9/1 -> Mux3/3
  Selector17/1 -> Sum13/1
  Sum13/1 -> H/1
  RwyElev/1 -> Sum13/2
  [gldN] -> Product4/2
  [locN] -> Product3/1
  Selector15/1 -> [gldN]
  Selector14/1 -> [locN]
  ILSnoise/1 -> Selector14/1, Selector15/1
  gldns/1 -> Product4/1
  Product4/1 -> Sum12/1
  Sum12/1 -> Mux1/2
  Product3/1 -> Sum10/1
  locns/1 -> Product3/2
  Sum10/1 -> Mux1/1
  Sum8/1 -> locns/1
  one/1 -> Sum8/1
  inv_xloc/1 -> Sum8/2
  Selector13/1 -> inv_xloc/1
  Gain1/1 -> Sat01/1
  Sum7/1 -> VzLG/1
  SlopeStart/1 -> Sum11/2
  Selector6/1 -> Mux3/1, Sum11/1
  Selector8/1 -> Mux3/2
  Mux3/1 -> xyzLG/1
  Sat/1 -> RwySlope2/1
  Product1/1 -> Sum7/1
  Sum11/1 -> Sat/1, Gain1/1
  RwySlope1/1 -> Product1/2
  Sat01/1 -> Product1/1
  Sum/1 -> Selector8/1, Selector3/1, Selector6/1
  X/1 -> Sum3/2, Sum/1, Selector17/1
  LG/1 -> Sum/2
  Sum4/1 -> Sum12/2
  tangGLD/1 -> Sum4/2
  Selector11/1 -> Sum4/1
  Selector12/1 -> Sum10/2
  Mux1/1 -> dyzILS/1
  xgld/1 -> Sum6/2
  Selector10/1 -> Sum6/1
  Sum6/1 -> tangGLD/1, gldns/1
  Sum3/1 -> Selector13/1, Selector12/1, Selector11/1, Selector10/1
  ILS/1 -> Sum3/1
  Lref1/1 -> ILS/1, LG/1
  Mux/1 -> Lref1/1
  "[dxGL  dzGL]"/1 -> Mux/6
  "[dxL  dzL]"/1 -> Mux/5
  "[dxLOC  dzLOC]"/1 -> Mux/4
  "[dxL   dzL]"/1 -> Mux/3
  "[dxGL   dzGL]"/1 -> Mux/2
  "[dxL dzL]"/1 -> Mux/1
  "[3 9]"/1 -> "[dxGL  dzGL]"/1, "[dxL  dzL]"/1
  Sum2/1 -> ssLG/1
  Selector9/1 -> Sum2/1
  PHI/1 -> Selector9/1
  "[2 8]"/1 -> "[dxLOC  dzLOC]"/1, "[dxL   dzL]"/1
  Sqrt/1 -> RwySlope1/1, Vground/1
  Selector7/1 -> Product2/1, Product2/2
  Selector4/1 -> Trigonometric Function/2
  Product2/1 -> Sqrt/1
  "[1 7]"/1 -> "[dxGL   dzGL]"/1, "[dxL dzL]"/1
  Trigonometric Function/1 -> Chi/1, Sum2/2
  Selector5/1 -> Trigonometric Function/1
  Selector1/1 -> Sum1/1
  [RV2B] -> "[2 8]"/1, "[3 9]"/1, "[1 7]"/1
  Sum1/1 -> Sum7/2, Vz/1
  Lref2/1 -> Sum1/2
  dxL/1 -> Lref2/1
  Selector2/1 -> dxL/1
  OM/1 -> Selector2/1
  Xdot/1 -> Selector7/1, Selector5/1, Selector4/1, Selector1/1

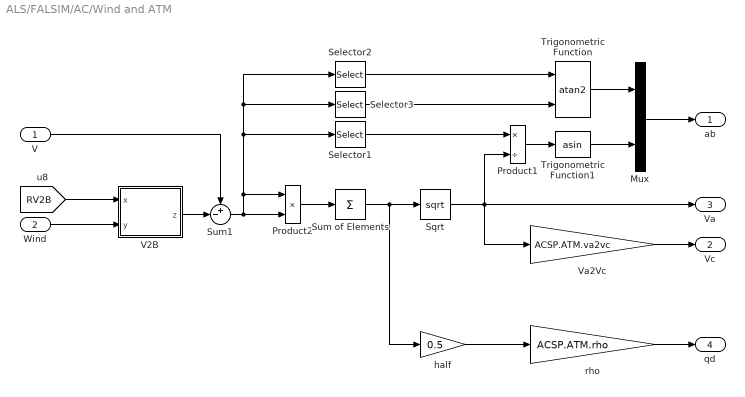
== system ALS/FALSIM/AC/Wind and ATM ==
  V : Inport
  Wind : Inport  Port=2
  Mux : Mux  Inputs=2
  Product1 : Product  Inputs=*/  SaturateOnIntegerOverflow=on  RndMeth=Zero  InputSameDT=on  OutDataTypeStr=Inherit: Same as first input
  Product2 : Product  SaturateOnIntegerOverflow=on  RndMeth=Zero  InputSameDT=on  OutDataTypeStr=Inherit: Same as first input
  Selector1 : Selector  InputPortWidth=3  IndexOptions=Index vector (dialog)  Indices=2  OutputSizes=1
  Selector2 : Selector  InputPortWidth=3  IndexOptions=Index vector (dialog)  Indices=3  OutputSizes=1
  Selector3 : Selector  InputPortWidth=3  IndexOptions=Index vector (dialog)  Indices=1  OutputSizes=1
  Sqrt : Sqrt  SaturateOnIntegerOverflow=on
  Sum of Elements : Sum  Inputs=+
  Sum1 : Sum  Inputs=+-|
  Trigonometric Function : Trigonometry  Operator=atan2
  Trigonometric Function1 : Trigonometry  Operator=asin
  V2B : Subsystem
      mask Display:
      | fprintf('MATRIX \n PRODUCT');
      | color('red');
      | fprintf('\n\n');
      | fprintf(' \n \n \n z=M(x)*y');
  Va2Vc : Gain  Gain=ACSP.ATM.va2vc
  half : Gain  Gain=0.5  SaturateOnIntegerOverflow=on  OutDataTypeStr=Inherit: Same as input  ParamDataTypeStr=Inherit: Same as input
  rho : Gain  Gain=ACSP.ATM.rho
  ab : Outport
  Vc : Outport  Port=2
  Va : Outport  Port=3
  qd : Outport  Port=4
  wires:
  Mux/1 -> ab/1
  Trigonometric Function1/1 -> Mux/2
  Trigonometric Function/1 -> Mux/1
  Sum of Elements/1 -> half/1, Sqrt/1
  Product1/1 -> Trigonometric Function1/1
  Sqrt/1 -> Va2Vc/1, Product1/2, Va/1
  Product2/1 -> Sum of Elements/1
  V/1 -> Sum1/1
  V2B/1(z) -> Sum1/2
  [RV2B] -> V2B/1(x)
  Selector3/1 -> Trigonometric Function/2
  Selector2/1 -> Trigonometric Function/1
  Selector1/1 -> Product1/1
  Sum1/1 -> Selector1/1, Selector2/1, Selector3/1, Product2/1, Product2/2
  Va2Vc/1 -> Vc/1
  half/1 -> rho/1
  rho/1 -> qd/1
  Wind/1 -> V2B/2(y)

== system ALS/FALSIM/Engines and Actuators/Actuators ==
  deltac : Inport
  Gain2 : Gain  Gain=1./ACSP.ACT.tau
  Int_ASD : Integrator  ContinuousStateAttributes='xASD'
  ML [55 25 30] : Saturate  UpperLimit=ACSP.ACT.ML  LowerLimit=-ACSP.ACT.ML
  RL [60 20 30] : Saturate  UpperLimit=ACSP.ACT.RL  LowerLimit=-ACSP.ACT.RL
  Sum : Sum  Inputs=|+-
  delta : Outport
  wires:
  Gain2/1 -> RL [60 20 30]/1
  RL [60 20 30]/1 -> Int_ASD/1
  Int_ASD/1 -> Sum/2, ML [55 25 30]/1
  deltac/1 -> Sum/1
  Sum/1 -> Gain2/1
  ML [55 25 30]/1 -> delta/1

== system ALS/FALSIM/Engines and Actuators/Engines ==
  epr0 : Inport
  eprc : Inport  Port=2
  EML : Saturate  UpperLimit=ACSP.ENG.UML  LowerLimit=ACSP.ENG.LML
  ERL : Saturate  UpperLimit=ACSP.ENG.RL  LowerLimit=-ACSP.ENG.RL
  Gain1 : Gain  Gain=1/ACSP.ENG.tau
  Gain2 : Gain  Gain=ACSP.ENG.Ga
  Gb : Constant  Value=ACSP.ENG.Gb
  Int_ENG : Integrator  ContinuousStateAttributes='xENG'
  Sum : Sum  Inputs=|+-
  Sum1 : Sum  Inputs=+-|
  Sum2 : Sum  Inputs=|++
  Sum3 : Sum  Inputs=++|
  TH : Outport
  epr : Outport  Port=2
  wires:
  Sum1/1 -> epr/1
  epr0/1 -> Sum2/2, Sum1/2
  EML/1 -> Gain2/1, Sum1/1
  Sum/1 -> Gain1/1
  Gain1/1 -> ERL/1
  ERL/1 -> Int_ENG/1
  Int_ENG/1 -> Sum/2, Sum2/1
  eprc/1 -> Sum/1
  Sum3/1 -> TH/1
  Gain2/1 -> Sum3/2
  Gb/1 -> Sum3/1
  Sum2/1 -> EML/1

== system ALS/FALSIM/AC/Dynamics/CP1 ==
  x : Inport
  y : Inport  Port=2
  Mux : Mux  Inputs=2
  Mux1 : Mux  Inputs=3
  Y1 : Fcn  Expr=u(2)*u(6)-u(3)*u(5)
  Y2 : Fcn  Expr=u(3)*u(4)-u(1)*u(6)
  Y3 : Fcn  Expr=u(1)*u(5)-u(2)*u(4)
  z : Outport
  wires:
  x/1 -> Mux/1
  Mux/1 -> Y1/1, Y3/1, Y2/1
  y/1 -> Mux/2
  Y3/1 -> Mux1/3
  Y1/1 -> Mux1/1
  Y2/1 -> Mux1/2
  Mux1/1 -> z/1

== system ALS/FALSIM/AC/Dynamics/CP2 ==
  x : Inport
  y : Inport  Port=2
  Mux : Mux  Inputs=2
  Mux1 : Mux  Inputs=3
  Y1 : Fcn  Expr=u(2)*u(6)-u(3)*u(5)
  Y2 : Fcn  Expr=u(3)*u(4)-u(1)*u(6)
  Y3 : Fcn  Expr=u(1)*u(5)-u(2)*u(4)
  z : Outport
  wires:
  x/1 -> Mux/1
  Mux/1 -> Y1/1, Y3/1, Y2/1
  y/1 -> Mux/2
  Y3/1 -> Mux1/3
  Y1/1 -> Mux1/1
  Y2/1 -> Mux1/2
  Mux1/1 -> z/1

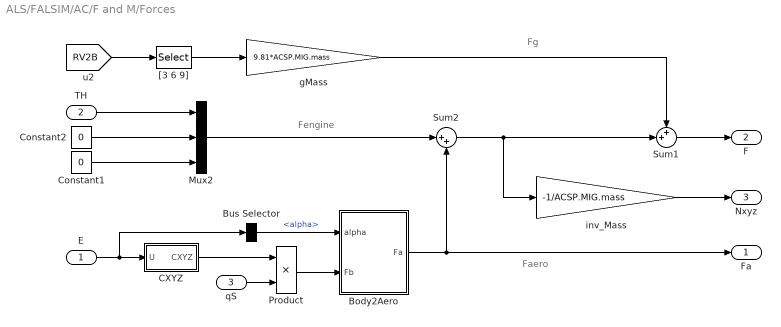
== system ALS/FALSIM/AC/F and M/Forces ==
  note: Faero
  note: Fengine
  note: Fg
  E : Inport
  TH : Inport  Port=2
  qS : Inport  Port=3
  Body2Aero : Subsystem
  Bus Selector : BusSelector  OutputSignals=alpha
  CXYZ : Subsystem
  Constant1 : Constant  Value=0
  Constant2 : Constant  Value=0
  Mux2 : Mux  Inputs=3
  Product : Product  RndMeth=Zero
  Sum1 : Sum  Inputs=++|
  Sum2 : Sum  Inputs=|++
  "[3 6 9]" : Selector  InputPortWidth=9  IndexOptions=Index vector (dialog)  Indices=[3 6 9]  OutputSizes=1
  gMass : Gain  Gain=9.81*ACSP.MIG.mass
  inv_Mass : Gain  Gain=-1/ACSP.MIG.mass
  Fa : Outport
  F : Outport  Port=2
  Nxyz : Outport  Port=3
  wires:
  TH/1 -> Mux2/1
  Constant2/1 -> Mux2/2
  Constant1/1 -> Mux2/3
  [RV2B] -> "[3 6 9]"/1
  "[3 6 9]"/1 -> gMass/1
  Sum1/1 -> F/1
  qS/1 -> Product/2
  Body2Aero/1(Fa) -> Sum2/2, Fa/1
  Product/1 -> Body2Aero/2(Fb)
  E/1 -> Bus Selector/1, CXYZ/1(U)
  CXYZ/1(CXYZ) -> Product/1
  Bus Selector/1 -> Body2Aero/1(alpha)  "<alpha>"
  Mux2/1 -> Sum2/1
  Sum2/1 -> inv_Mass/1, Sum1/2
  gMass/1 -> Sum1/1
  inv_Mass/1 -> Nxyz/1

== system ALS/FALSIM/AC/F and M/Moments ==
  note: MFaero
  note: Mengine
  note: Ma
  E : Inport
  Fa : Inport  Port=2
  qS : Inport  Port=3
  TH : Inport  Port=4
  CD0 : Constant  Value=ACSP.MIG.dxG
  CP : Subsystem
      mask Display:
      | fprintf('CROSS \n PRODUCT');
      | color('red');
      | fprintf('\n\n');
      | fprintf(' \n \n \n z=x^y');
      | %text(3,1,'PRODUCT');
      | %text(5,1,'z=x^y');
  Clmn : Subsystem
  Constant{1..4} (4 alike) : Constant  Value=0
  Engine vertical position : Gain  Gain=ACSP.MIG.dzE
  Lref : Gain  Gain=ACSP.MIG.Lref
  Mux1 : Mux  Inputs=3
  Mux2 : Mux  Inputs=3
  Product : Product  RndMeth=Zero
  Sum1 : Sum  Inputs=+++
  M : Outport
  wires:
  Constant1/1 -> Mux2/3
  Sum1/1 -> Lref/1
  TH/1 -> Engine vertical position/1
  Engine vertical position/1 -> Mux2/2
  Constant2/1 -> Mux2/1
  qS/1 -> Product/1
  Fa/1 -> CP/2(y)
  Mux1/1 -> CP/1(x)
  CP/1(z) -> Sum1/1
  Constant3/1 -> Mux1/2
  Constant4/1 -> Mux1/3
  CD0/1 -> Mux1/1
  Product/1 -> Sum1/2
  Mux2/1 -> Sum1/3
  Lref/1 -> M/1
  Clmn/1(Clmn) -> Product/2
  E/1 -> Clmn/1(U)

== system ALS/FALSIM/AC/Kinematics/R(PHI) ==
  x : Inport
  y : Inport  Port=2
  Mux : Mux  Inputs=2
  Mux1 : Mux  Inputs=3
  Y1 : Fcn  Expr=u(1)*u(10)+u(2)*u(11)+u(3)*u(12)
  Y2 : Fcn  Expr=u(4)*u(10)+u(5)*u(11)+u(6)*u(12)
  Y3 : Fcn  Expr=u(7)*u(10)+u(8)*u(11)+u(9)*u(12)
  z : Outport
  wires:
  x/1 -> Mux/1
  Mux/1 -> Y3/1, Y1/1, Y2/1
  y/1 -> Mux/2
  Y3/1 -> Mux1/3
  Y1/1 -> Mux1/1
  Y2/1 -> Mux1/2
  Mux1/1 -> z/1

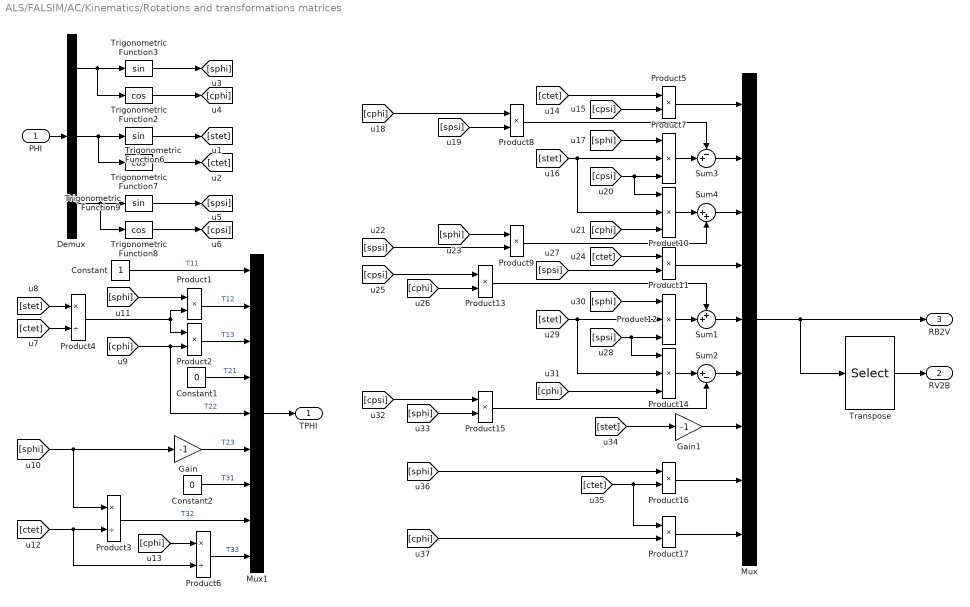
== system ALS/FALSIM/AC/Kinematics/Rotations and transformations matrices ==
  PHI : Inport
  Constant : Constant
  Constant1 : Constant  Value=0
  Constant2 : Constant  Value=0
  Demux : Demux  Outputs=3
  Gain : Gain  Gain=-1
  Gain1 : Gain  Gain=-1
  Mux : Mux  Inputs=9
  Mux1 : Mux  Inputs=9
  Product{1..2,5,8..9,11,13,15..17} (10 alike) : Product  SaturateOnIntegerOverflow=on  RndMeth=Zero  InputSameDT=on  OutDataTypeStr=Inherit: Same as first input
  Product{7,10,12,14} (4 alike) : Product  Inputs=3  SaturateOnIntegerOverflow=on  RndMeth=Zero  InputSameDT=on  OutDataTypeStr=Inherit: Same as first input
  Product3 : Product  Inputs=*/  SaturateOnIntegerOverflow=on  RndMeth=Zero  InputSameDT=on  OutDataTypeStr=Inherit: Same as first input
  Product4 : Product  Inputs=*/  SaturateOnIntegerOverflow=on  RndMeth=Zero  InputSameDT=on  OutDataTypeStr=Inherit: Same as first input
  Product6 : Product  Inputs=*/  SaturateOnIntegerOverflow=on  RndMeth=Zero  InputSameDT=on  OutDataTypeStr=Inherit: Same as first input
  Sum1 : Sum  Inputs=++|
  Sum2 : Sum  Inputs=|+-
  Sum3 : Sum  Inputs=-+|
  Sum4 : Sum  Inputs=|++
  Transpose : Selector  InputPortWidth=9  IndexOptions=Index vector (dialog)  Indices=[1 4 7 2 5 8 3 6 9]  OutputSizes=1
  Trigonometric Function2 : Trigonometry  Operator=cos
  Trigonometric Function3 : Trigonometry
  Trigonometric Function6 : Trigonometry
  Trigonometric Function7 : Trigonometry  Operator=cos
  Trigonometric Function8 : Trigonometry  Operator=cos
  Trigonometric Function9 : Trigonometry
  TPHI : Outport
  RV2B : Outport  Port=2
  RB2V : Outport  Port=3
  wires:
  [stet] -> Product4/1
  [ctet] -> Product4/2
  [sphi] -> Product1/1
  Product4/1 -> Product1/2, Product2/1
  Trigonometric Function8/1 -> [cpsi]
  Trigonometric Function9/1 -> [spsi]
  Demux/3 -> Trigonometric Function9/1, Trigonometric Function8/1
  Trigonometric Function6/1 -> [stet]
  Trigonometric Function7/1 -> [ctet]
  Demux/2 -> Trigonometric Function7/1, Trigonometric Function6/1
  Trigonometric Function2/1 -> [cphi]
  Demux/1 -> Trigonometric Function3/1, Trigonometric Function2/1
  Trigonometric Function3/1 -> [sphi]
  [cphi] -> Mux1/5, Product2/2  "T22"
  Product1/1 -> Mux1/2  "T12"
  [ctet] -> Product6/2, Product3/2
  Constant/1 -> Mux1/1  "T11"
  Product2/1 -> Mux1/3  "T13"
  Constant1/1 -> Mux1/4  "T21"
  Product6/1 -> Mux1/9  "T33"
  [sphi] -> Product3/1, Gain/1
  Constant2/1 -> Mux1/7  "T31"
  Gain/1 -> Mux1/6  "T23"
  [cphi] -> Product6/1
  Product3/1 -> Mux1/8  "T32"
  PHI/1 -> Demux/1
  Product5/1 -> Mux/1
  [ctet] -> Product5/1
  [cpsi] -> Product5/2
  [stet] -> Product10/2, Product7/2
  [cphi] -> Product8/1
  [spsi] -> Product8/2
  Product7/1 -> Sum3/2
  Sum3/1 -> Mux/2
  Product8/1 -> Sum3/1
  Sum4/1 -> Mux/3
  Product10/1 -> Sum4/1
  [sphi] -> Product7/1
  [cpsi] -> Product10/1, Product7/3
  [cphi] -> Product10/3
  Product9/1 -> Sum4/2
  [sphi] -> Product9/1
  [spsi] -> Product9/2
  [ctet] -> Product11/1
  Product11/1 -> Mux/4
  Product12/1 -> Sum1/2
  Sum1/1 -> Mux/5
  [cpsi] -> Product13/1
  [cphi] -> Product13/2
  Product13/1 -> Sum1/1
  [spsi] -> Product11/2
  [spsi] -> Product14/1, Product12/3
  [stet] -> Product14/2, Product12/2
  [sphi] -> Product12/1
  Product14/1 -> Sum2/1
  Sum2/1 -> Mux/6
  [cphi] -> Product14/3
  [cpsi] -> Product15/1
  [sphi] -> Product15/2
  Product15/1 -> Sum2/2
  Gain1/1 -> Mux/7
  [stet] -> Gain1/1
  Product16/1 -> Mux/8
  [ctet] -> Product17/1, Product16/2
  Product17/1 -> Mux/9
  [sphi] -> Product16/1
  [cphi] -> Product17/2
  Mux1/1 -> TPHI/1
  Mux/1 -> Transpose/1, RB2V/1
  Transpose/1 -> RV2B/1

== system ALS/FALSIM/AC/Kinematics/T(PHI) ==
  x : Inport
  y : Inport  Port=2
  Mux : Mux  Inputs=2
  Mux1 : Mux  Inputs=3
  Y1 : Fcn  Expr=u(1)*u(10)+u(2)*u(11)+u(3)*u(12)
  Y2 : Fcn  Expr=u(4)*u(10)+u(5)*u(11)+u(6)*u(12)
  Y3 : Fcn  Expr=u(7)*u(10)+u(8)*u(11)+u(9)*u(12)
  z : Outport
  wires:
  x/1 -> Mux/1
  Mux/1 -> Y3/1, Y1/1, Y2/1
  y/1 -> Mux/2
  Y3/1 -> Mux1/3
  Y1/1 -> Mux1/1
  Y2/1 -> Mux1/2
  Mux1/1 -> z/1

== system ALS/FALSIM/AC/Wind and ATM/V2B ==
  x : Inport
  y : Inport  Port=2
  Mux : Mux  Inputs=2
  Mux1 : Mux  Inputs=3
  Y1 : Fcn  Expr=u(1)*u(10)+u(2)*u(11)+u(3)*u(12)
  Y2 : Fcn  Expr=u(4)*u(10)+u(5)*u(11)+u(6)*u(12)
  Y3 : Fcn  Expr=u(7)*u(10)+u(8)*u(11)+u(9)*u(12)
  z : Outport
  wires:
  x/1 -> Mux/1
  Mux/1 -> Y3/1, Y1/1, Y2/1
  y/1 -> Mux/2
  Y3/1 -> Mux1/3
  Y1/1 -> Mux1/1
  Y2/1 -> Mux1/2
  Mux1/1 -> z/1

== system ALS/FALSIM/AC/F and M/Forces/Body2Aero ==
  alpha : Inport
  Fb : Inport  Port=2
  Fy : Selector  InputPortWidth=5  IndexOptions=Index vector (dialog)  Indices=4  OutputSizes=1
  Mux : Mux  Inputs=[1 1 3]
  Mux3 : Mux  Inputs=3
  Trigonometric Function1 : Trigonometry
  Trigonometric Function2 : Trigonometry  Operator=cos
  ca*Fx-sa*Fz : Fcn  Expr=u(1)*u(3)-u(2)*u(5)
  sa*Fx+ca*Fz : Fcn  Expr=u(2)*u(3)+u(1)*u(5)
  Fa : Outport
  wires:
  alpha/1 -> Trigonometric Function1/1, Trigonometric Function2/1
  Fb/1 -> Mux/3
  Trigonometric Function1/1 -> Mux/2
  Trigonometric Function2/1 -> Mux/1
  sa*Fx+ca*Fz/1 -> Mux3/3
  ca*Fx-sa*Fz/1 -> Mux3/1
  Mux/1 -> sa*Fx+ca*Fz/1, ca*Fx-sa*Fz/1, Fy/1
  Mux3/1 -> Fa/1
  Fy/1 -> Mux3/2

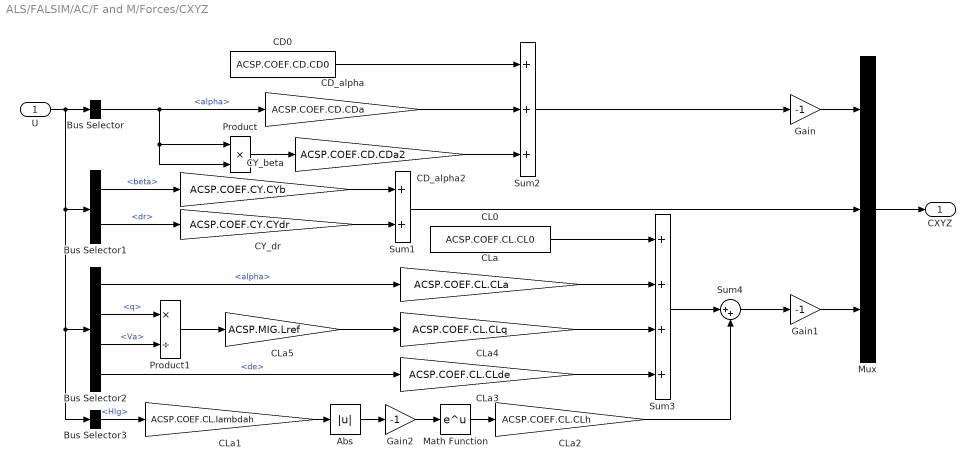
== system ALS/FALSIM/AC/F and M/Forces/CXYZ ==
  U : Inport
  Abs : Abs
  Bus Selector : BusSelector  OutputSignals=alpha
  Bus Selector1 : BusSelector  OutputSignals=beta,dr
  Bus Selector2 : BusSelector  OutputSignals=alpha,q,Va,de
  Bus Selector3 : BusSelector  OutputSignals=Hlg
  CD0 : Constant  Value=ACSP.COEF.CD.CD0
  CD_alpha : Gain  Gain=ACSP.COEF.CD.CDa
  CD_alpha2 : Gain  Gain=ACSP.COEF.CD.CDa2
  CL0 : Constant  Value=ACSP.COEF.CL.CL0
  CLa : Gain  Gain=ACSP.COEF.CL.CLa
  CLa1 : Gain  Gain=ACSP.COEF.CL.lambdah
  CLa2 : Gain  Gain=ACSP.COEF.CL.CLh
  CLa3 : Gain  Gain=ACSP.COEF.CL.CLde
  CLa4 : Gain  Gain=ACSP.COEF.CL.CLq
  CLa5 : Gain  Gain=ACSP.MIG.Lref
  CY_beta : Gain  Gain=ACSP.COEF.CY.CYb
  CY_dr : Gain  Gain=ACSP.COEF.CY.CYdr
  Gain : Gain  Gain=-1
  Gain1 : Gain  Gain=-1
  Gain2 : Gain  Gain=-1
  Math Function : Math  SaturateOnIntegerOverflow=on
  Mux : Mux  Inputs=3
  Product : Product  RndMeth=Zero
  Product1 : Product  Inputs=*/  RndMeth=Zero
  Sum1 : Sum
  Sum2 : Sum  Inputs=+++
  Sum3 : Sum  Inputs=++++
  Sum4 : Sum  Inputs=|++
  CXYZ : Outport
  wires:
  CLa5/1 -> CLa4/1
  U/1 -> Bus Selector3/1, Bus Selector2/1, Bus Selector1/1, Bus Selector/1
  Bus Selector/1 -> Product/2, Product/1, CD_alpha/1  "<alpha>"
  Product/1 -> CD_alpha2/1
  Bus Selector1/1 -> CY_beta/1  "<beta>"
  Bus Selector1/2 -> CY_dr/1  "<dr>"
  CY_beta/1 -> Sum1/1
  CY_dr/1 -> Sum1/2
  CD_alpha/1 -> Sum2/2
  CD_alpha2/1 -> Sum2/3
  CD0/1 -> Sum2/1
  CLa1/1 -> Abs/1
  Gain2/1 -> Math Function/1
  Abs/1 -> Gain2/1
  Math Function/1 -> CLa2/1
  Product1/1 -> CLa5/1
  CLa/1 -> Sum3/2
  Bus Selector2/2 -> Product1/1  "<q>"
  Bus Selector2/3 -> Product1/2  "<Va>"
  Bus Selector2/1 -> CLa/1  "<alpha>"
  CL0/1 -> Sum3/1
  Gain1/1 -> Mux/3
  Gain/1 -> Mux/1
  Sum1/1 -> Mux/2
  Mux/1 -> CXYZ/1
  Bus Selector2/4 -> CLa3/1  "<de>"
  CLa3/1 -> Sum3/4
  Sum3/1 -> Sum4/1
  Bus Selector3/1 -> CLa1/1  "<Hlg>"
  CLa2/1 -> Sum4/2
  CLa4/1 -> Sum3/3
  Sum2/1 -> Gain/1
  Sum4/1 -> Gain1/1

== system ALS/FALSIM/AC/F and M/Moments/CP ==
  x : Inport
  y : Inport  Port=2
  Mux : Mux  Inputs=2
  Mux1 : Mux  Inputs=3
  Y1 : Fcn  Expr=u(2)*u(6)-u(3)*u(5)
  Y2 : Fcn  Expr=u(3)*u(4)-u(1)*u(6)
  Y3 : Fcn  Expr=u(1)*u(5)-u(2)*u(4)
  z : Outport
  wires:
  x/1 -> Mux/1
  Mux/1 -> Y1/1, Y3/1, Y2/1
  y/1 -> Mux/2
  Y3/1 -> Mux1/3
  Y1/1 -> Mux1/1
  Y2/1 -> Mux1/2
  Mux1/1 -> z/1

== system ALS/FALSIM/AC/F and M/Moments/Clmn ==
  U : Inport
  Cl : Subsystem
  Cm : Subsystem
  Cn : Subsystem
  Mux : Mux  Inputs=3
  Clmn : Outport
  wires:
  U/1 -> Cn/1(U), Cl/1(U), Cm/1(U)
  Cl/1(Cl) -> Mux/1
  Cm/1(Cm) -> Mux/2
  Cn/1(Cn) -> Mux/3
  Mux/1 -> Clmn/1

== system ALS/FALSIM/AC/F and M/Moments/Clmn/Cl ==
  U : Inport
  Bus Selector : BusSelector  OutputSignals=beta,p,alpha,r,Va,da,dr
  CD0 : Constant  Value=ACSP.COEF.Cl.Clr0
  CD_alpha : Gain  Gain=ACSP.COEF.Cl.Clb
  CD_alpha1 : Gain  Gain=ACSP.COEF.Cl.Clp
  CD_alpha2 : Gain  Gain=ACSP.COEF.Cl.Clra
  CD_alpha3 : Gain  Gain=ACSP.COEF.Cl.Clda
  CD_alpha4 : Gain  Gain=ACSP.COEF.Cl.Cldr
  CLa3 : Gain  Gain=ACSP.MIG.Lref
  Product1 : Product  RndMeth=Zero
  Product2 : Product  Inputs=*/  RndMeth=Zero
  Sum1 : Sum
  Sum2 : Sum  Inputs=+++
  Sum4 : Sum  Inputs=|++
  Sum5 : Sum  Inputs=++|
  Cl : Outport
  wires:
  U/1 -> Bus Selector/1
  Bus Selector/3 -> CD_alpha2/1  "<alpha>"
  Bus Selector/4 -> Product1/2  "<r>"
  Bus Selector/6 -> CD_alpha3/1  "<da>"
  Product1/1 -> Sum5/2
  CD_alpha1/1 -> Sum5/1
  Bus Selector/7 -> CD_alpha4/1  "<dr>"
  Product2/1 -> CLa3/1
  Sum4/1 -> Product1/1
  CD_alpha/1 -> Sum2/1
  CD_alpha3/1 -> Sum1/1
  Bus Selector/1 -> CD_alpha/1  "<beta>"
  CD_alpha2/1 -> Sum4/1
  CD_alpha4/1 -> Sum1/2
  Sum2/1 -> Cl/1
  Bus Selector/2 -> CD_alpha1/1  "<p>"
  Bus Selector/5 -> Product2/2  "<Va>"
  Sum1/1 -> Sum2/3
  CLa3/1 -> Sum2/2
  Sum5/1 -> Product2/1
  CD0/1 -> Sum4/2

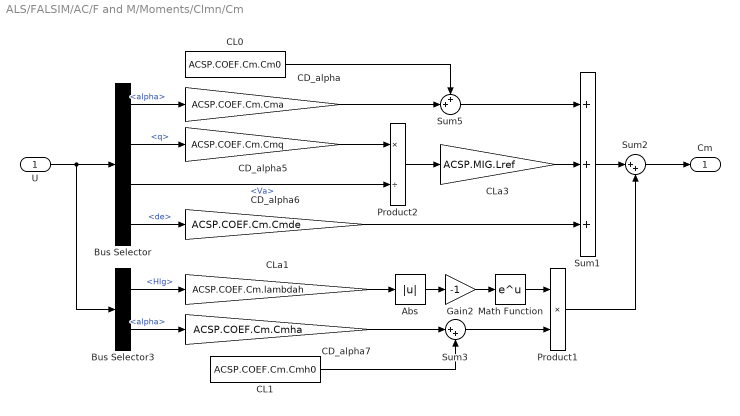
== system ALS/FALSIM/AC/F and M/Moments/Clmn/Cm ==
  U : Inport
  Abs : Abs
  Bus Selector : BusSelector  OutputSignals=alpha,q,Va,de
  Bus Selector3 : BusSelector  OutputSignals=Hlg,alpha
  CD_alpha : Gain  Gain=ACSP.COEF.Cm.Cma
  CD_alpha5 : Gain  Gain=ACSP.COEF.Cm.Cmq
  CD_alpha6 : Gain  Gain=ACSP.COEF.Cm.Cmde
  CD_alpha7 : Gain  Gain=ACSP.COEF.Cm.Cmha
  CL0 : Constant  Value=ACSP.COEF.Cm.Cm0
  CL1 : Constant  Value=ACSP.COEF.Cm.Cmh0
  CLa1 : Gain  Gain=ACSP.COEF.Cm.lambdah
  CLa3 : Gain  Gain=ACSP.MIG.Lref
  Gain2 : Gain  Gain=-1
  Math Function : Math  SaturateOnIntegerOverflow=on
  Product1 : Product  RndMeth=Zero
  Product2 : Product  Inputs=*/  RndMeth=Zero
  Sum1 : Sum  Inputs=+++
  Sum2 : Sum  Inputs=|++
  Sum3 : Sum  Inputs=|++
  Sum5 : Sum  Inputs=++|
  Cm : Outport
  wires:
  U/1 -> Bus Selector3/1, Bus Selector/1
  Bus Selector/1 -> CD_alpha/1  "<alpha>"
  Bus Selector/2 -> CD_alpha5/1  "<q>"
  CD_alpha5/1 -> Product2/1
  Bus Selector/3 -> Product2/2  "<Va>"
  Product2/1 -> CLa3/1
  Bus Selector/4 -> CD_alpha6/1  "<de>"
  CLa1/1 -> Abs/1
  Gain2/1 -> Math Function/1
  Abs/1 -> Gain2/1
  Sum1/1 -> Sum2/1
  Product1/1 -> Sum2/2
  Math Function/1 -> Product1/1
  Bus Selector3/1 -> CLa1/1  "<Hlg>"
  Bus Selector3/2 -> CD_alpha7/1  "<alpha>"
  CD_alpha7/1 -> Sum3/1
  CL1/1 -> Sum3/2
  Sum3/1 -> Product1/2
  CD_alpha/1 -> Sum5/2
  CL0/1 -> Sum5/1
  CD_alpha6/1 -> Sum1/3
  CLa3/1 -> Sum1/2
  Sum5/1 -> Sum1/1
  Sum2/1 -> Cm/1

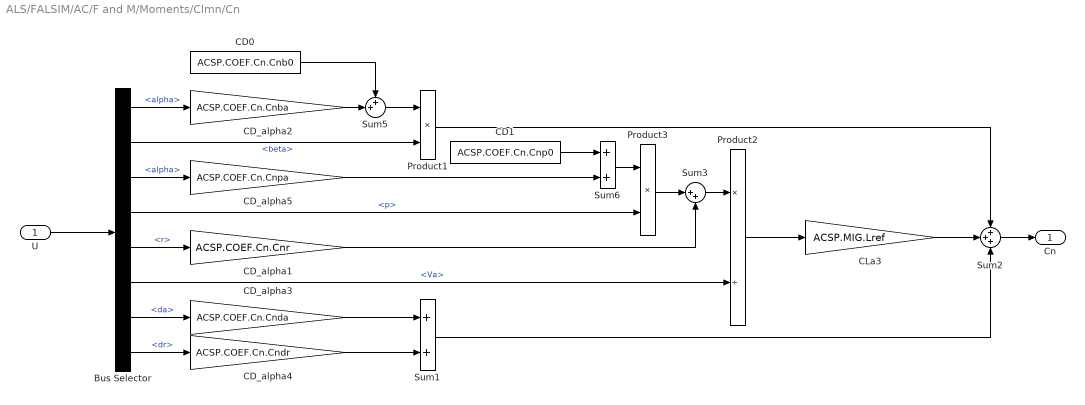
== system ALS/FALSIM/AC/F and M/Moments/Clmn/Cn ==
  U : Inport
  Bus Selector : BusSelector  OutputSignals=alpha,beta,alpha,p,r,Va,da,dr
  CD0 : Constant  Value=ACSP.COEF.Cn.Cnb0
  CD1 : Constant  Value=ACSP.COEF.Cn.Cnp0
  CD_alpha1 : Gain  Gain=ACSP.COEF.Cn.Cnr
  CD_alpha2 : Gain  Gain=ACSP.COEF.Cn.Cnba
  CD_alpha3 : Gain  Gain=ACSP.COEF.Cn.Cnda
  CD_alpha4 : Gain  Gain=ACSP.COEF.Cn.Cndr
  CD_alpha5 : Gain  Gain=ACSP.COEF.Cn.Cnpa
  CLa3 : Gain  Gain=ACSP.MIG.Lref
  Product1 : Product  RndMeth=Zero
  Product2 : Product  Inputs=*/  RndMeth=Zero
  Product3 : Product  RndMeth=Zero
  Sum1 : Sum
  Sum2 : Sum  Inputs=+++
  Sum3 : Sum  Inputs=|++
  Sum5 : Sum  Inputs=++|
  Sum6 : Sum
  Cn : Outport
  wires:
  U/1 -> Bus Selector/1
  Product2/1 -> CLa3/1
  Sum2/1 -> Cn/1
  Bus Selector/1 -> CD_alpha2/1  "<alpha>"
  CD_alpha2/1 -> Sum5/2
  CD0/1 -> Sum5/1
  Bus Selector/2 -> Product1/2  "<beta>"
  Sum5/1 -> Product1/1
  Bus Selector/3 -> CD_alpha5/1  "<alpha>"
  Product1/1 -> Sum2/1
  CD_alpha5/1 -> Sum6/2
  CD1/1 -> Sum6/1
  Sum6/1 -> Product3/1
  Bus Selector/4 -> Product3/2  "<p>"
  Bus Selector/5 -> CD_alpha1/1  "<r>"
  CD_alpha1/1 -> Sum3/2
  Bus Selector/6 -> Product2/2  "<Va>"
  Bus Selector/7 -> CD_alpha3/1  "<da>"
  Bus Selector/8 -> CD_alpha4/1  "<dr>"
  CD_alpha3/1 -> Sum1/1
  CD_alpha4/1 -> Sum1/2
  Sum1/1 -> Sum2/3
  CLa3/1 -> Sum2/2
  Product3/1 -> Sum3/1
  Sum3/1 -> Product2/1
